simulink model "sf_abs"  (Simulink 7.6)
settings: Solver=VariableStepDiscrete  StartTime=0.0  StopTime=20  MaxStep=.2  RelTol=1e-3
settings Model: Creator=The MathWorks Inc.  ExtModeAutoUpdateStatusClock=off
settings SolverCC: ZeroCrossControl=EnableAll  InsertRTBMode=Auto
settings OptimizationCC: InitFltsAndDblsToZero=on
settings DebuggingCC: SignalResolutionControl=TryResolveAllWithWarning  StrictBusMsg=Warning
settings SFSimCC: SFSimEnableDebug=off  SFSimOverflowDetection=off  SFSimEcho=off  SimParseCustomCode=off
settings GRTTargetCC: TargetFcnLib=ansi_tfl_tmw_new.mat

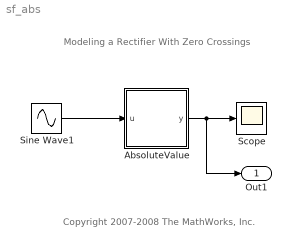
== system sf_abs ==
  note: Modeling a Rectifier With Zero Crossings
  note: Copyright 2007-2008 The MathWorks, Inc.
  AbsoluteValue : Stateflow chart  TreatAsAtomicUnit=on
  Scope : Scope
  Sine Wave1 : Sin  SampleTime=0
  Out1 : Outport
  wires:
  AbsoluteValue/1(y) -> Scope/1, Out1/1
  Sine Wave1/1 -> AbsoluteValue/1(u)

== stateflow chart AbsoluteValue ==
  settings: updateMethod=CONTINUOUS
  state P
    du: y = u;
  state N
    du: y = -u;
  P -> N : [u < 0]
  N -> P : [u >= 0]
  (default) -> (junction 5)
  (junction 5) -> P [order 1] : [u >= 0]
  (junction 5) -> (junction 6) [order 2]
  (junction 6) -> N
  data: u input double; y output double
